simulink model "demostration"  (R2014b)
settings: Solver=ode45  StartTime=0.0  StopTime=10.0  RelTol=1e-3
settings Model: Creator=wangze  LastModifiedBy=wangze

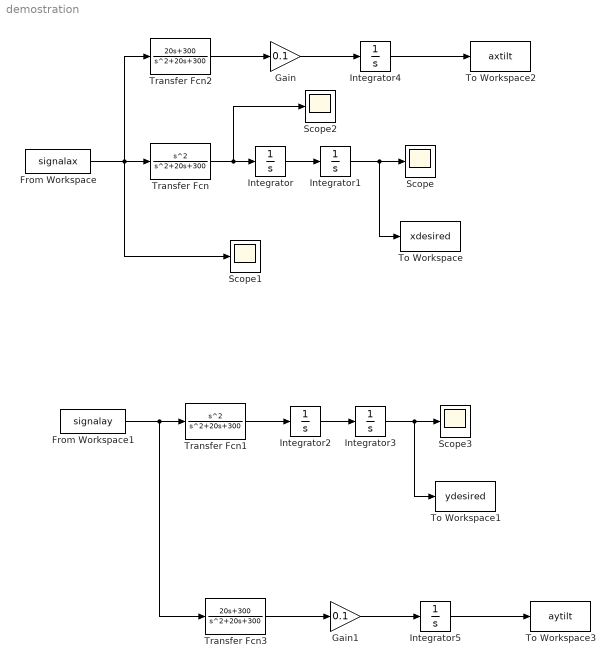
== system demostration ==
  From Workspace : FromWorkspace  VariableName=signalax  SampleTime=0.05
  From Workspace1 : FromWorkspace  VariableName=signalay  SampleTime=0
  Gain : Gain  Gain=0.1
  Gain1 : Gain  Gain=0.1
  Integrator{,1..5} (6 alike) : Integrator
  Scope{,1..3} (4 alike) : Scope
      Scope2 settings: SaveName=ScopeData2
      Scope3 settings: SaveName=ScopeData3
  To Workspace : ToWorkspace  VariableName=xdesired  SampleTime=0.05
      settings: Decimation=2  Save2DSignal=2-D array (concatenate along first dimension)
  To Workspace1 : ToWorkspace  VariableName=ydesired  SampleTime=0.05
      settings: Decimation=2  Save2DSignal=2-D array (concatenate along first dimension)
  To Workspace2 : ToWorkspace  VariableName=axtilt  SampleTime=-1
      settings: Decimation=2
  To Workspace3 : ToWorkspace  VariableName=aytilt  SampleTime=-1
      settings: Decimation=2
  Transfer Fcn : TransferFcn  Numerator=[1 0 0]  Denominator=[1 20 300]
  Transfer Fcn1 : TransferFcn  Numerator=[1 0 0]  Denominator=[1 20 300]
  Transfer Fcn2 : TransferFcn  Numerator=[20 300]  Denominator=[1 20 300]
  Transfer Fcn3 : TransferFcn  Numerator=[20 300]  Denominator=[1 20 300]
  wires:
  From Workspace/1 -> Transfer Fcn2/1, Scope1/1, Transfer Fcn/1
  Transfer Fcn/1 -> Scope2/1, Integrator/1
  Integrator/1 -> Integrator1/1
  Integrator1/1 -> To Workspace/1, Scope/1
  From Workspace1/1 -> Transfer Fcn1/1, Transfer Fcn3/1
  Transfer Fcn1/1 -> Integrator2/1
  Integrator2/1 -> Integrator3/1
  Integrator3/1 -> Scope3/1, To Workspace1/1
  Transfer Fcn2/1 -> Gain/1
  Integrator4/1 -> To Workspace2/1
  Gain/1 -> Integrator4/1
  Integrator5/1 -> To Workspace3/1
  Gain1/1 -> Integrator5/1
  Transfer Fcn3/1 -> Gain1/1
